simulink model "car_navigation_model"  (R2015a)
settings: Solver=ode3  StartTime=0.0  StopTime=200  FixedStep=0.01  RelTol=1e-3
libraries: simulink x8, fuzblock x1
settings Model: Creator=ALKATRAZ  LastModifiedBy=ALKATRAZ

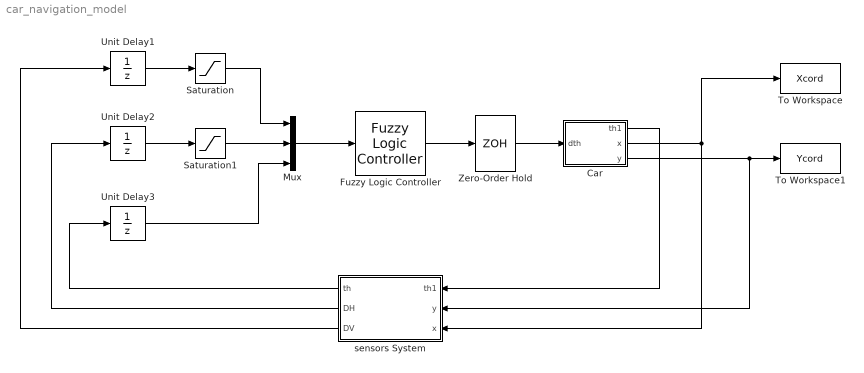
== system car_navigation_model ==
  Car : Subsystem
  Fuzzy Logic Controller : fuzblock/Fuzzy Logic  Controller  fis='FLCFinal.fis'
  Mux : Mux  Inputs=3
  Saturation : Saturate  UpperLimit=1  LowerLimit=0
  Saturation1 : Saturate  UpperLimit=1  LowerLimit=0
  To Workspace : ToWorkspace  VariableName=Xcord  SaveFormat=Timeseries  SampleTime=-1
  To Workspace1 : ToWorkspace  VariableName=Ycord  SaveFormat=Timeseries  SampleTime=-1
  Unit Delay1 : UnitDelay  SampleTime=0.01
  Unit Delay2 : UnitDelay  SampleTime=0.01
  Unit Delay3 : UnitDelay  SampleTime=0.01
  Zero-Order Hold : ZeroOrderHold  SampleTime=0.01
  sensors System : Subsystem
  wires:
  sensors System/2(DH) -> Unit Delay2/1
  Fuzzy Logic Controller/1 -> Zero-Order Hold/1
  Zero-Order Hold/1 -> Car/1(dth)
  Car/2(x) -> To Workspace/1, sensors System/3(x)
  Car/3(y) -> sensors System/2(y), To Workspace1/1
  Unit Delay2/1 -> Saturation1/1
  Unit Delay3/1 -> Mux/3
  Car/1(th1) -> sensors System/1(th1)
  sensors System/1(th) -> Unit Delay3/1
  Mux/1 -> Fuzzy Logic Controller/1
  Saturation/1 -> Mux/1
  Saturation1/1 -> Mux/2
  sensors System/3(DV) -> Unit Delay1/1
  Unit Delay1/1 -> Saturation/1

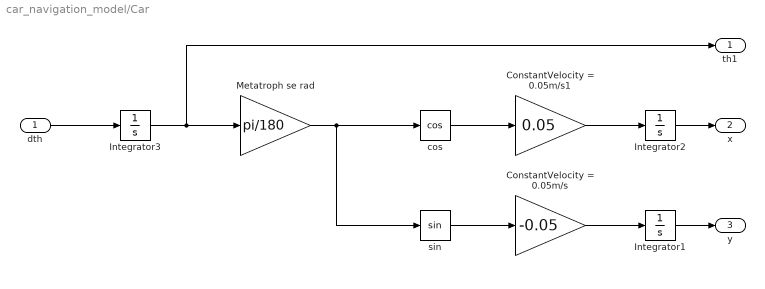
== system car_navigation_model/Car ==
  dth : Inport
  " sin" : Trigonometry
  ConstantVelocity = 0.05m/s : Gain  Gain=-0.05
  ConstantVelocity = 0.05m/s1 : Gain  Gain=0.05
  Integrator1 : Integrator  InitialCondition=4.3
  Integrator2 : Integrator  InitialCondition=9.1
  Integrator3 : Integrator  InitialCondition=90
  Metatroph se rad : Gain  Gain=pi/180
  "cos " : Trigonometry  Operator=cos
  th1 : Outport
  x : Outport  Port=2
  y : Outport  Port=3
  wires:
  Integrator3/1 -> th1/1, Metatroph se rad/1
  dth/1 -> Integrator3/1
  Metatroph se rad/1 -> "cos "/1, " sin"/1
  " sin"/1 -> ConstantVelocity = 0.05m/s/1
  ConstantVelocity = 0.05m/s/1 -> Integrator1/1
  Integrator1/1 -> y/1
  "cos "/1 -> ConstantVelocity = 0.05m/s1/1
  Integrator2/1 -> x/1
  ConstantVelocity = 0.05m/s1/1 -> Integrator2/1

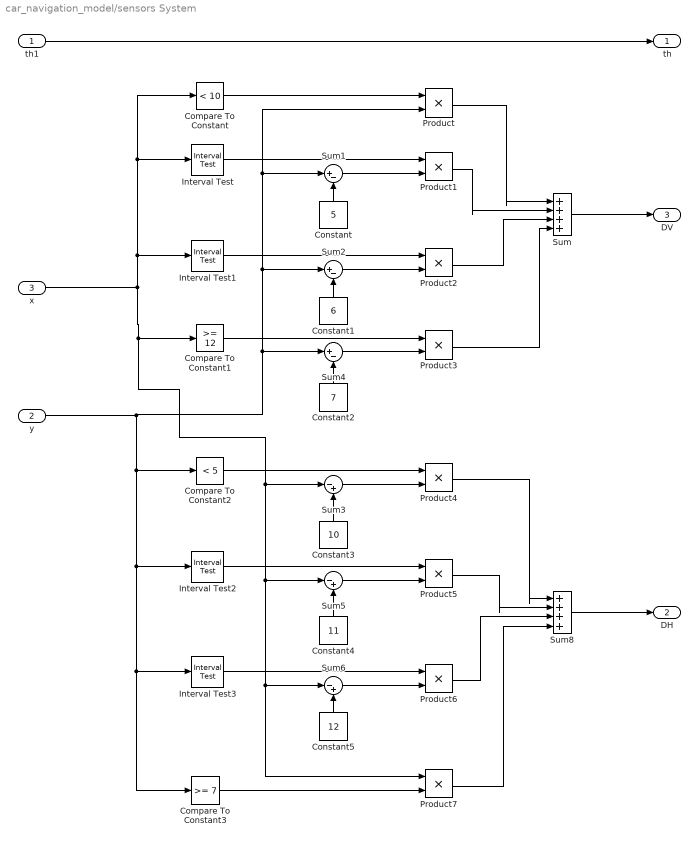
== system car_navigation_model/sensors System ==
  th1 : Inport
  y : Inport  Port=2
  x : Inport  Port=3
  Compare To Constant : simulink/Logic and Bit Operations/Compare To Constant  relop=<  const=10  OutDataTypeStr=boolean
  Compare To Constant1 : simulink/Logic and Bit Operations/Compare To Constant  relop=>=  const=12  OutDataTypeStr=boolean
  Compare To Constant2 : simulink/Logic and Bit Operations/Compare To Constant  relop=<  const=5  OutDataTypeStr=boolean
  Compare To Constant3 : simulink/Logic and Bit Operations/Compare To Constant  relop=>=  const=7  OutDataTypeStr=boolean
  Constant : Constant  Value=5
  Constant1 : Constant  Value=6
  Constant2 : Constant  Value=7
  Constant3 : Constant  Value=10
  Constant4 : Constant  Value=11
  Constant5 : Constant  Value=12
  Interval Test : simulink/Logic and Bit Operations/Interval Test  IntervalClosedRight=off  uplimit=11  IntervalClosedLeft=on  lowlimit=10  OutDataTypeStr=boolean
  Interval Test1 : simulink/Logic and Bit Operations/Interval Test  IntervalClosedRight=off  uplimit=12  IntervalClosedLeft=on  lowlimit=11  OutDataTypeStr=boolean
  Interval Test2 : simulink/Logic and Bit Operations/Interval Test  IntervalClosedRight=off  uplimit=6  IntervalClosedLeft=on  lowlimit=5  OutDataTypeStr=boolean
  Interval Test3 : simulink/Logic and Bit Operations/Interval Test  IntervalClosedRight=off  uplimit=7  IntervalClosedLeft=on  lowlimit=6  OutDataTypeStr=boolean
  Product{,1..7} (8 alike) : Product
  Sum : Sum  Inputs=|++++
  Sum1 : Sum  Inputs=|+-
  Sum2 : Sum  Inputs=|+-
  Sum3 : Sum  Inputs=|-+
  Sum4 : Sum  Inputs=|+-
  Sum5 : Sum  Inputs=|-+
  Sum6 : Sum  Inputs=|-+
  Sum8 : Sum  Inputs=|++++
  th : Outport
  DH : Outport  Port=2
  DV : Outport  Port=3
  wires:
  Compare To Constant/1 -> Product/1
  Product/1 -> Sum/1
  Compare To Constant1/1 -> Product3/1
  Product1/1 -> Sum/2
  Constant1/1 -> Sum2/2
  y/1 -> Sum4/1, Sum2/1, Sum1/1, Product/2, Compare To Constant3/1, Interval Test3/1, Interval Test2/1, Compare To Constant2/1
  Constant2/1 -> Sum4/2
  Compare To Constant2/1 -> Product4/1
  Compare To Constant3/1 -> Product7/2
  Constant3/1 -> Sum3/2
  x/1 -> Sum3/1, Sum5/1, Product7/1, Sum6/1, Compare To Constant1/1, Interval Test/1, Compare To Constant/1, Interval Test1/1
  Constant4/1 -> Sum5/2
  Constant5/1 -> Sum6/2
  th1/1 -> th/1
  Sum8/1 -> DH/1
  Sum/1 -> DV/1
  Constant/1 -> Sum1/2
  Interval Test/1 -> Product1/1
  Sum1/1 -> Product1/2
  Interval Test1/1 -> Product2/1
  Sum2/1 -> Product2/2
  Sum4/1 -> Product3/2
  Product2/1 -> Sum/3
  Product3/1 -> Sum/4
  Sum3/1 -> Product4/2
  Sum5/1 -> Product5/2
  Interval Test2/1 -> Product5/1
  Interval Test3/1 -> Product6/1
  Sum6/1 -> Product6/2
  Product4/1 -> Sum8/1
  Product5/1 -> Sum8/2
  Product6/1 -> Sum8/3
  Product7/1 -> Sum8/4
